simulink model "uav_control_fb_lil_pp"  (R2023a)
settings: Solver=FixedStepAuto  StartTime=0.0  StopTime=50  FixedStep=1e-3
undefined symbols (not defined in the file): b, d, g, J1, J2, J3, K, L, m, Matrix_Force2angular_velocity
libraries: simulink x22, hamilton x1, lagrange x1, control_form_NL x1, control_form_NL_forces x1
(part 2 of 2)

== matlab function uav_control_fb_lil_pp/MATLAB Function ==
  data: x input; delta_inv output; y input; z input; phi input; theta input; psi input; xdot input; ydot input; zdot input; zeta input; xi input; p input; q input; r input
function delta_inv = delta_inv_function(x,y,z,phi,theta,psi,xdot,ydot,zdot,zeta,xi,p,q,r)

% prep
m=1.88;
g=9.81;
J1=1.453e-2;
J2=1.453e-2;
J3=2.884e-2;

input1=0;
input2=0;
input3=0;
input4=0;

sphi=sin(phi);
cphi=cos(phi);
stheta=sin(theta);
ctheta=cos(theta);
spsi=sin(psi);
cpsi=cos(psi);

% model dynamics
phi_dot=p+q*(sin(phi)*tan(theta))+r*(cos(phi)*tan(theta));
theta_dot=q*cos(phi)-r*sin(phi);
psi_dot=q*sin(phi)/cos(theta)+r*cos(phi)/cos(theta);


zeta_dot=xi;
xi_dot=input1;

p_dot=(J2-J3)/J1*q*r+1/J1*input2;
q_dot=(J3-J1)/J2*r*p+1/J2*input3;
r_dot=(J1-J2)/J3*p*q+1/J3*input4;

%others
phi_d_dot=p_dot+q_dot*sphi*tan(theta)+phi_dot*q*cphi*tan(theta)+theta_dot*q*sphi/(ctheta^2)+...
r_dot*cphi*tan(theta)-phi_dot*r*sphi*tan(theta)+theta_dot*r*cphi/(ctheta^2);

theta_d_dot=q_dot*cphi-phi_dot*q*sphi-r_dot*sphi-r*phi_dot*cphi;

psi_d_dot=q_dot*sphi/ctheta+q/(ctheta^2)*(phi_dot*cphi*ctheta+theta_dot*sphi*stheta)+...
r_dot*cphi/ctheta+r/(ctheta^2)*(-phi_dot*sphi*ctheta+theta_dot*cphi*stheta);

%%%--------------------------------------------------------------------------------------

%x

Cx=cphi*stheta*cpsi+sphi*spsi;

Cx_dot=-phi_dot*sphi*stheta*cpsi+theta_dot*cphi*ctheta*cpsi-psi_dot*cphi*stheta*spsi...
+phi_dot*cphi*spsi+psi_dot*sphi*cpsi;

Cx_d_dot=psi_d_dot*(-sphi*stheta*cpsi+cphi*spsi)+theta_d_dot*cphi*ctheta*cpsi...
+psi_d_dot*(-cphi*stheta*spsi+sphi*cpsi)-cphi*stheta*cpsi*(phi_dot^2+theta_dot^2+psi_dot^2)...
-2*phi_dot*theta_dot*sphi*ctheta*cpsi+2*phi_dot*psi_dot*sphi*stheta*spsi...
-2*theta_dot*psi_dot*cphi*ctheta*spsi-sphi*spsi*(phi_dot^2+psi_dot^2)+2*phi_dot*psi_dot*cphi*cpsi;

x_4dots=-1/m*(input1*Cx+2*xi*Cx_dot+zeta*Cx_d_dot); % Lf4h1(x)
LgLf3h1=-1/m*[Cx,...
    1/J1*zeta*(-sphi*stheta*cpsi+cphi*spsi),...
    1/J2*zeta*((-sphi*stheta*cpsi+cphi*spsi)*sphi*tan(theta)+cphi*ctheta*cpsi*cphi+...
    (-cphi*stheta*spsi+sphi*cpsi)*sphi/ctheta),...
    1/J3*zeta*((-sphi*stheta*cpsi+cphi*spsi)*cphi*tan(theta)-cphi*ctheta*cpsi*sphi+...
    (-cphi*stheta*spsi+sphi*cpsi)*cphi/ctheta)];

%y

Cy=cphi*stheta*spsi-sphi*cpsi;

Cy_dot=-phi_dot*sphi*stheta*spsi+theta_dot*cphi*ctheta*spsi+psi_dot*cphi*stheta*cpsi...
-phi_dot*cphi*cpsi+psi_dot*sphi*spsi;

Cy_d_dot=phi_d_dot*(-sphi*stheta*spsi-cphi*cpsi)+theta_d_dot*cphi*ctheta*spsi...
+psi_d_dot*(cphi*stheta*cpsi+sphi*spsi)-cphi*stheta*spsi*(phi_dot^2+theta_dot^2+psi_dot^2)...
-2*phi_dot*theta_dot*sphi*ctheta*spsi-2*phi_dot*psi_dot*sphi*stheta*cpsi...
+2*theta_dot*psi_dot*cphi*ctheta*cpsi+sphi*cpsi*(phi_dot^2+psi_dot^2)+2*phi_dot*psi_dot*cphi*spsi;

y_4dots=-1/m*(input1*Cy+2*xi*Cy_dot+zeta*Cy_d_dot);
LgLf3h2=-1/m*[Cy,...
    1/J1*zeta*(-sphi*stheta*spsi-cphi*cpsi),...
    1/J2*zeta*((-sphi*stheta*spsi-cphi*cpsi)*sphi*tan(theta)+cphi*ctheta*spsi*cphi+...
    (cphi*stheta*cpsi+sphi*spsi)*sphi/ctheta),...
    1/J3*zeta*((-sphi*stheta*spsi-cphi*cpsi)*cphi*tan(theta)-cphi*ctheta*spsi*sphi+...
    (cphi*stheta*cpsi+sphi*spsi)*cphi/ctheta)];
%z
Cz=cphi*ctheta;

Cz_dot=-phi_dot*sphi*ctheta-theta_dot*cphi*stheta;

Cz_d_dot=-phi_d_dot*sphi*ctheta-phi_dot^2*cphi*ctheta+2*phi_dot*theta_dot*sphi*stheta...
    -theta_d_dot*cphi*stheta-theta_dot^2*cphi*ctheta;

z_4dots=-1/m*(input1*Cz+2*xi*Cz_dot+zeta*Cz_d_dot);
LgLf3h3=-1/m*[Cz,...
    1/J1*zeta*(-sphi*ctheta),...
    1/J2*zeta*(-sphi*ctheta*sphi*tan(theta)-cphi*stheta*cphi),...
    1/J3*zeta*(-sphi*ctheta*cphi*tan(theta)+cphi*stheta*sphi)];

%psi

%psi_d_dot is defined above
LgLf1h4=[0,...
    0,...
    1/J2*sphi/ctheta,...
    1/J3*cphi/ctheta];
delta_inv = inv([LgLf3h1;LgLf3h2;LgLf3h3;LgLf1h4]);

== matlab function uav_control_fb_lil_pp/MATLAB Function2 ==
  data: x input; transf output; y input; z input; phi input; theta input; psi input; xdot input; ydot input; zdot input; zeta input; xi input; p input; q input; r input
function transf = transform_difeo_function(x,y,z,phi,theta,psi,xdot,ydot,zdot,zeta,xi,p,q,r)

% prep
m=1.88;
g=9.81;
J1=1.453e-2;
J2=1.453e-2;
J3=2.884e-2;

input1=0;
input2=0;
input3=0;
input4=0;

sphi=sin(phi);
cphi=cos(phi);
stheta=sin(theta);
ctheta=cos(theta);
spsi=sin(psi);
cpsi=cos(psi);

% model dynamics
phi_dot=p+q*(sin(phi)*tan(theta))+r*(cos(phi)*tan(theta));
theta_dot=q*cos(phi)-r*sin(phi);
psi_dot=q*sin(phi)/cos(theta)+r*cos(phi)/cos(theta);


zeta_dot=xi;
xi_dot=input1;

p_dot=(J2-J3)/J1*q*r+1/J1*input2;
q_dot=(J3-J1)/J2*r*p+1/J2*input3;
r_dot=(J1-J2)/J3*p*q+1/J3*input4;

%others
phi_d_dot=p_dot+q_dot*sphi*tan(theta)+phi_dot*q*cphi*tan(theta)+theta_dot*q*sphi/(ctheta^2)+...
r_dot*cphi*tan(theta)-phi_dot*r*sphi*tan(theta)+theta_dot*r*cphi/(ctheta^2);

theta_d_dot=q_dot*cphi-phi_dot*q*sphi-r_dot*sphi-r*phi_dot*cphi;

psi_d_dot=q_dot*sphi/ctheta+q/(ctheta^2)*(phi_dot*cphi*ctheta+theta_dot*sphi*stheta)+...
r_dot*cphi/ctheta+r/(ctheta^2)*(-phi_dot*sphi*ctheta+theta_dot*cphi*stheta);

%%%--------------------------------------------------------------------------------------

%x

Cx=cphi*stheta*cpsi+sphi*spsi;

Cx_dot=-phi_dot*sphi*stheta*cpsi+theta_dot*cphi*ctheta*cpsi-psi_dot*cphi*stheta*spsi...
+phi_dot*cphi*spsi+psi_dot*sphi*cpsi;

Cx_d_dot=psi_d_dot*(-sphi*stheta*cpsi+cphi*spsi)+theta_d_dot*cphi*ctheta*cpsi...
+psi_d_dot*(-cphi*stheta*spsi+sphi*cpsi)-cphi*stheta*cpsi*(phi_dot^2+theta_dot^2+psi_dot^2)...
-2*phi_dot*theta_dot*sphi*ctheta*cpsi+2*phi_dot*psi_dot*sphi*stheta*spsi...
-2*theta_dot*psi_dot*cphi*ctheta*spsi-sphi*spsi*(phi_dot^2+psi_dot^2)+2*phi_dot*psi_dot*cphi*cpsi;

x_4dots=-1/m*(input1*Cx+2*xi*Cx_dot+zeta*Cx_d_dot); % Lf4h1(x)
LgLf3h1=-1/m*[Cx,...
    1/J1*zeta*(-sphi*stheta*cpsi+cphi*spsi),...
    1/J2*zeta*((-sphi*stheta*cpsi+cphi*spsi)*sphi*tan(theta)+cphi*ctheta*cpsi*cphi+...
    (-cphi*stheta*spsi+sphi*cpsi)*sphi/ctheta),...
    1/J3*zeta*((-sphi*stheta*cpsi+cphi*spsi)*cphi*tan(theta)-cphi*ctheta*cpsi*sphi+...
    (-cphi*stheta*spsi+sphi*cpsi)*cphi/ctheta)];

Lf0h1=x;
Lf1h1=xdot;
Lf2h1=-1/m*zeta*Cx;
Lf3h1=-1/m*(xi*Cx+zeta*Cx_dot);

%y

Cy=cphi*stheta*spsi-sphi*cpsi;

Cy_dot=-phi_dot*sphi*stheta*spsi+theta_dot*cphi*ctheta*spsi+psi_dot*cphi*stheta*cpsi...
-phi_dot*cphi*cpsi+psi_dot*sphi*spsi;

Cy_d_dot=phi_d_dot*(-sphi*stheta*spsi-cphi*cpsi)+theta_d_dot*cphi*ctheta*spsi...
+psi_d_dot*(cphi*stheta*cpsi+sphi*spsi)-cphi*stheta*spsi*(phi_dot^2+theta_dot^2+psi_dot^2)...
-2*phi_dot*theta_dot*sphi*ctheta*spsi-2*phi_dot*psi_dot*sphi*stheta*cpsi...
+2*theta_dot*psi_dot*cphi*ctheta*cpsi+sphi*cpsi*(phi_dot^2+psi_dot^2)+2*phi_dot*psi_dot*cphi*spsi;

y_4dots=-1/m*(input1*Cy+2*xi*Cy_dot+zeta*Cy_d_dot);
LgLf3h2=-1/m*[Cy,...
    1/J1*zeta*(-sphi*stheta*spsi-cphi*cpsi),...
    1/J2*zeta*((-sphi*stheta*spsi-cphi*cpsi)*sphi*tan(theta)+cphi*ctheta*spsi*cphi+...
    (cphi*stheta*cpsi+sphi*spsi)*sphi/ctheta),...
    1/J3*zeta*((-sphi*stheta*spsi-cphi*cpsi)*cphi*tan(theta)-cphi*ctheta*spsi*sphi+...
    (cphi*stheta*cpsi+sphi*spsi)*cphi/ctheta)];

Lf0h2=y;
Lf1h2=ydot;
Lf2h2=-1/m*zeta*Cy;
Lf3h2=-1/m*(xi*Cy+zeta*Cy_dot);

%z
Cz=cphi*ctheta;

Cz_dot=-phi_dot*sphi*ctheta-theta_dot*cphi*stheta;

Cz_d_dot=-phi_d_dot*sphi*ctheta-phi_dot^2*cphi*ctheta+2*phi_dot*theta_dot*sphi*stheta...
    -theta_d_dot*cphi*stheta-theta_dot^2*cphi*ctheta;

z_4dots=-1/m*(input1*Cz+2*xi*Cz_dot+zeta*Cz_d_dot);
LgLf3h3=-1/m*[Cz,...
    1/J1*zeta*(-sphi*ctheta),...
    1/J2*zeta*(-sphi*ctheta*sphi*tan(theta)-cphi*stheta*cphi),...
    1/J3*zeta*(-sphi*ctheta*cphi*tan(theta)+cphi*stheta*sphi)];

Lf0h3=z;
Lf1h3=zdot;
Lf2h3=g-1/m*zeta*Cz;
Lf3h3=-1/m*(xi*Cz+zeta*Cz_dot);
%psi
Lf0h4=psi;
Lf1h4=psi_dot;
%psi_d_dot is defined above
LgLf1h4=[0,...
    0,...
    1/J2*sphi/ctheta,...
    1/J3*cphi/ctheta];
transf=[Lf0h1,Lf1h1,Lf2h1,Lf3h1,Lf0h2,Lf1h2,Lf2h2,Lf3h2,Lf0h3,Lf1h3,Lf2h3,Lf3h3,Lf0h4,Lf1h4]';
